simulink model "gm_HDL_pfc_gold_fi_vnl"  (R2024b)
settings: Solver=FixedStepDiscrete  StartTime=0.0  StopTime=.4  RelTol=1e-3
InitFcn:
  | fidelity_pfc_vals;
  | load('C:\Users\Angel\Desktop\hil\pfc3ph\matlab\sim\sschdl\pfc_desktop\stateSpaceParameters.mat');
undefined symbols (not defined in the file or in its folder): a, b, c, DiscIntNeverNeededParam, Down, Gs, s, stateSpaceParameters_1, t_ss, tsw, Up
libraries: simulink x32, hdlmdlgenlib x24, hdlsllib x8, eePwmGenerator x3, dspsrcs4 x3, hdlssclib x2, simulink_need_slupdate x1
(part 2 of 4)

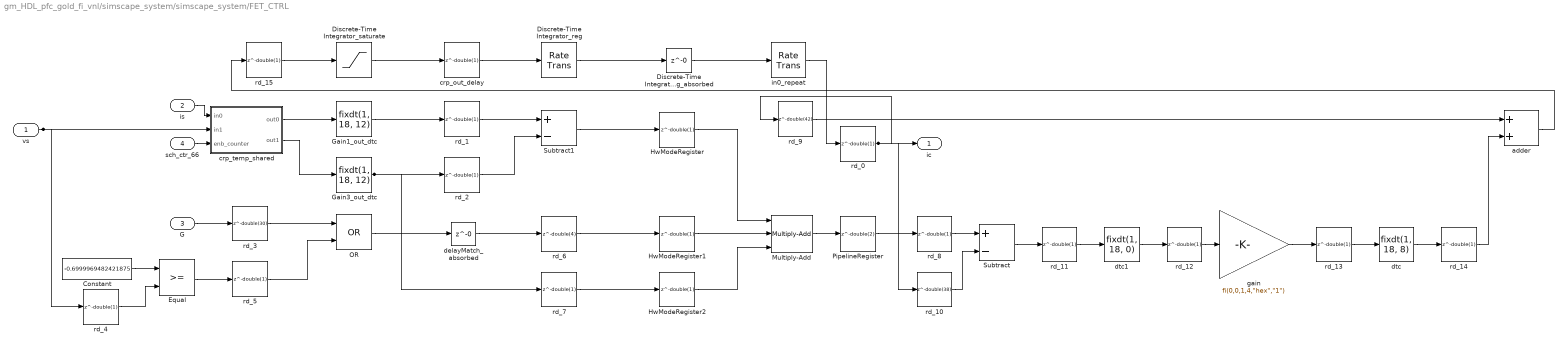
== system gm_HDL_pfc_gold_fi_vnl/simscape_system/simscape_system/FET_CTRL ==
  vs : Inport  OutDataTypeStr=fixdt(1, 18, 6)  PortDimensions=[6]  SampleTime=7.65403750478377e-09
  is : Inport  Port=2  OutDataTypeStr=fixdt(1, 18, 6)  PortDimensions=[6]  SampleTime=7.65403750478377e-09
  G : Inport  Port=3  OutDataTypeStr=boolean  PortDimensions=[6]  SampleTime=7.65403750478377e-09
  sch_ctr_66 : Inport  Port=4  OutDataTypeStr=fixdt(0, 7, 0)  SampleTime=7.65403750478377e-09
  Constant : Constant  Value=-0.6999969482421875  OutDataTypeStr=fixdt(1, 18, 17)  SampleTime=7.65403750478377e-09
  Discrete-Time Integrator_reg : RateTransition  InitialCondition=double(0)  OutPortSampleTimeOpt=Multiple of input port sample time  OutPortSampleTimeMultiple=67
  Discrete-Time Integrator_reg_absorbed : Delay  DelayLength=0
  Discrete-Time Integrator_saturate : Saturate  UpperLimit="fi(0,1,18,8,\"hex\",\"06400\")"  LowerLimit="fi(0,1,18,8,\"hex\",\"39c00\")"  SampleTime=7.65403750478377e-09  OutDataTypeStr=fixdt(1, 18, 8)
  Equal : RelationalOperator  OutDataTypeStr=boolean  SampleTime=7.65403750478377e-09  InputSameDT=off
  Gain1_out_dtc : DataTypeConversion  OutDataTypeStr=fixdt(1, 18, 12)  SampleTime=7.65403750478377e-09  SaturateOnIntegerOverflow=off  RndMeth=Floor
  Gain3_out_dtc : DataTypeConversion  OutDataTypeStr=fixdt(1, 18, 12)  SampleTime=7.65403750478377e-09  SaturateOnIntegerOverflow=off  RndMeth=Floor
  HwModeRegister : Delay  DelayLength=double(1)  InitialCondition=0  SampleTime=7.65403750478377e-09
  HwModeRegister1 : Delay  DelayLength=double(1)  InitialCondition=0  SampleTime=7.65403750478377e-09
  HwModeRegister2 : Delay  DelayLength=double(1)  InitialCondition=0  SampleTime=7.65403750478377e-09
  Multiply-Add : hdlsllib/HDL Operations/Multiply-Add  Function=c+(a.*b)  datatype=fixdt(1, 18, 12)  DoSatur=on  FMA=off
  OR : Logic  Operator=OR  AllPortsSameDT=off  OutDataTypeStr=boolean  SampleTime=7.65403750478377e-09
  PipelineRegister : Delay  DelayLength=double(2)  InitialCondition=0  SampleTime=7.65403750478377e-09
  Subtract : Sum  Inputs=+-  OutDataTypeStr=fixdt(1, 18, 12)  AccumDataTypeStr=fixdt(1, 23, 12)  SampleTime=7.65403750478377e-09
  Subtract1 : Sum  Inputs=+-  OutDataTypeStr=fixdt(1, 18, 11)  AccumDataTypeStr=fixdt(1, 19, 12)  SampleTime=7.65403750478377e-09
  adder : Sum  OutDataTypeStr=fixdt(1, 18, 8)  AccumDataTypeStr=fixdt(1, 18, 8)  SaturateOnIntegerOverflow=on  SampleTime=7.65403750478377e-09
  crp_out_delay : Delay  DelayLength=double(1)  InitialCondition=0  SampleTime=7.65403750478377e-09
  crp_temp_shared : Subsystem
  delayMatch_absorbed : Delay  DelayLength=0
  dtc : DataTypeConversion  OutDataTypeStr=fixdt(1, 18, 8)  ConvertRealWorld=Stored Integer (SI)  SampleTime=7.65403750478377e-09  RndMeth=Floor
  dtc1 : DataTypeConversion  OutDataTypeStr=fixdt(1, 18, 0)  ConvertRealWorld=Stored Integer (SI)  SampleTime=7.65403750478377e-09  RndMeth=Floor
  gain : Gain  Gain="fi(0,0,1,4,\"hex\",\"1\")"  ParamDataTypeStr=fixdt(0, 1, 4)  OutDataTypeStr=fixdt(1, 18, 0)  SaturateOnIntegerOverflow=on  SampleTime=7.65403750478377e-09
  in0_repeat : RateTransition  Integrity=off  Deterministic=off  OutPortSampleTimeOpt=Multiple of input port sample time  OutPortSampleTimeMultiple=1/67
  rd_{0..2,4..5,7..8,11..15} (12 alike) : Delay  DelayLength=double(1)  InitialCondition=0  SampleTime=7.65403750478377e-09
  rd_10 : Delay  DelayLength=double(38)  InitialCondition=0  SampleTime=7.65403750478377e-09
  rd_3 : Delay  DelayLength=double(30)  InitialCondition=0  SampleTime=7.65403750478377e-09
  rd_6 : Delay  DelayLength=double(4)  InitialCondition=0  SampleTime=7.65403750478377e-09
  rd_9 : Delay  DelayLength=double(42)  InitialCondition=0  SampleTime=7.65403750478377e-09
  ic : Outport  SampleTime=7.65403750478377e-09
  wires:
  adder/1 -> rd_15/1
  rd_14/1 -> adder/2
  rd_13/1 -> dtc/1
  dtc1/1 -> rd_12/1
  rd_8/1 -> Subtract/1
  PipelineRegister/1 -> rd_8/1
  rd_9/1 -> adder/1
  in0_repeat/1 -> rd_0/1
  HwModeRegister1/1 -> Multiply-Add/2
  rd_0/1 -> ic/1, rd_10/1, rd_9/1
  HwModeRegister/1 -> Multiply-Add/1
  Discrete-Time Integrator_reg_absorbed/1 -> in0_repeat/1
  gain/1 -> rd_13/1
  rd_7/1 -> HwModeRegister2/1
  rd_6/1 -> HwModeRegister1/1
  Multiply-Add/1 -> PipelineRegister/1
  delayMatch_absorbed/1 -> rd_6/1
  rd_2/1 -> Subtract1/2
  Discrete-Time Integrator_reg/1 -> Discrete-Time Integrator_reg_absorbed/1
  rd_1/1 -> Subtract1/1
  Subtract1/1 -> HwModeRegister/1
  crp_out_delay/1 -> Discrete-Time Integrator_reg/1
  Gain3_out_dtc/1 -> rd_2/1, rd_7/1
  Gain1_out_dtc/1 -> rd_1/1
  rd_11/1 -> dtc1/1
  Discrete-Time Integrator_saturate/1 -> crp_out_delay/1
  rd_5/1 -> OR/2
  dtc/1 -> rd_14/1
  rd_3/1 -> OR/1
  crp_temp_shared/2(out1) -> Gain3_out_dtc/1
  OR/1 -> delayMatch_absorbed/1
  Subtract/1 -> rd_11/1
  crp_temp_shared/1(out0) -> Gain1_out_dtc/1
  Equal/1 -> rd_5/1
  is/1 -> crp_temp_shared/1(in0)
  sch_ctr_66/1 -> crp_temp_shared/3(enb_counter)
  G/1 -> rd_3/1
  rd_12/1 -> gain/1
  rd_4/1 -> Equal/2
  Constant/1 -> Equal/1
  HwModeRegister2/1 -> Multiply-Add/3
  rd_15/1 -> Discrete-Time Integrator_saturate/1
  vs/1 -> rd_4/1, crp_temp_shared/2(in1)
  rd_10/1 -> Subtract/2

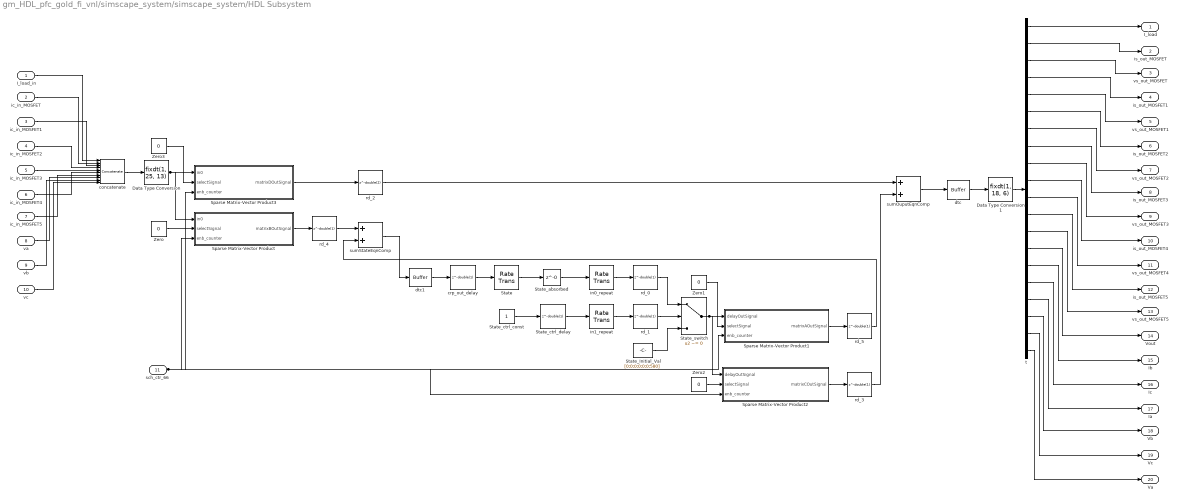
== system gm_HDL_pfc_gold_fi_vnl/simscape_system/simscape_system/HDL Subsystem ==
  I_load_in : Inport  OutDataTypeStr=fixdt(1, 18, 8)  PortDimensions=1  SampleTime=7.65403750478377e-09
  ic_in_MOSFET : Inport  Port=2  OutDataTypeStr=fixdt(1, 18, 8)  PortDimensions=1  SampleTime=7.65403750478377e-09
  ic_in_MOSFET1 : Inport  Port=3  OutDataTypeStr=fixdt(1, 18, 8)  PortDimensions=1  SampleTime=7.65403750478377e-09
  ic_in_MOSFET2 : Inport  Port=4  OutDataTypeStr=fixdt(1, 18, 8)  PortDimensions=1  SampleTime=7.65403750478377e-09
  ic_in_MOSFET3 : Inport  Port=5  OutDataTypeStr=fixdt(1, 18, 8)  PortDimensions=1  SampleTime=7.65403750478377e-09
  ic_in_MOSFET4 : Inport  Port=6  OutDataTypeStr=fixdt(1, 18, 8)  PortDimensions=1  SampleTime=7.65403750478377e-09
  ic_in_MOSFET5 : Inport  Port=7  OutDataTypeStr=fixdt(1, 18, 8)  PortDimensions=1  SampleTime=7.65403750478377e-09
  va : Inport  Port=8  OutDataTypeStr=fixdt(1, 18, 8)  PortDimensions=1  SampleTime=7.65403750478377e-09
  vb : Inport  Port=9  OutDataTypeStr=fixdt(1, 18, 8)  PortDimensions=1  SampleTime=7.65403750478377e-09
  vc : Inport  Port=10  OutDataTypeStr=fixdt(1, 18, 8)  PortDimensions=1  SampleTime=7.65403750478377e-09
  sch_ctr_66 : Inport  Port=11  OutDataTypeStr=fixdt(0, 7, 0)  SampleTime=7.65403750478377e-09
  Data Type Conversion : DataTypeConversion  OutDataTypeStr=fixdt(1, 25, 13)  SampleTime=7.65403750478377e-09  SaturateOnIntegerOverflow=off  RndMeth=Floor
  Data Type Conversion1 : DataTypeConversion  OutDataTypeStr=fixdt(1, 18, 6)  SampleTime=7.65403750478377e-09  SaturateOnIntegerOverflow=off  RndMeth=Floor
  Sparse Matrix-Vector Product : Subsystem
  Sparse Matrix-Vector Product1 : Subsystem
  Sparse Matrix-Vector Product2 : Subsystem
  Sparse Matrix-Vector Product3 : Subsystem
  State : RateTransition  InitialCondition=double(0)  OutPortSampleTimeOpt=Multiple of input port sample time  OutPortSampleTimeMultiple=67
  State_Initial_Val : Constant  Value=[0;0;0;0;0;0;580]  OutDataTypeStr=fixdt(1, 25, 13)  SampleTime=7.65403750478377e-09
  State_absorbed : Delay  DelayLength=0
  State_ctrl_const : Constant  OutDataTypeStr=boolean  SampleTime=5.12820512820513e-07
  State_ctrl_delay : Delay  DelayLength=double(1)  InitialCondition=0  SampleTime=5.12820512820513e-07
  State_switch : Switch  Criteria=u2 ~= 0  Threshold=double(0)  OutDataTypeStr=fixdt(1, 25, 13)  SampleTime=7.65403750478377e-09  SaturateOnIntegerOverflow=off  InputSameDT=off
  Zero{,1..3} (4 alike) : Constant  Value=0  OutDataTypeStr=boolean  SampleTime=7.65403750478377e-09
  concatenate : Concatenate  NumInputs=10
  crp_out_delay : Delay  DelayLength=double(1)  InitialCondition=0  SampleTime=7.65403750478377e-09
  dtc : hdlmdlgenlib/Buffer
  dtc1 : hdlmdlgenlib/Buffer
  in0_repeat : RateTransition  Integrity=off  Deterministic=off  OutPortSampleTimeOpt=Multiple of input port sample time  OutPortSampleTimeMultiple=1/67
  in1_repeat : RateTransition  Integrity=off  Deterministic=off  OutPortSampleTimeOpt=Multiple of input port sample time  OutPortSampleTimeMultiple=1/67
  rd_{0..1,3..5} (5 alike) : Delay  DelayLength=double(1)  InitialCondition=0  SampleTime=7.65403750478377e-09
  rd_2 : Delay  DelayLength=double(2)  InitialCondition=0  SampleTime=7.65403750478377e-09
  sumOuputEqnComp : Sum  OutDataTypeStr=fixdt(1, 25, 13)  SampleTime=7.65403750478377e-09
  sumStateEqnComp : Sum  OutDataTypeStr=fixdt(1, 25, 13)  SampleTime=7.65403750478377e-09
  t : Demux  Outputs=20
  I_load : Outport  SampleTime=7.65403750478377e-09
  is_out_MOSFET : Outport  Port=2  SampleTime=7.65403750478377e-09
  vs_out_MOSFET : Outport  Port=3  SampleTime=7.65403750478377e-09
  is_out_MOSFET1 : Outport  Port=4  SampleTime=7.65403750478377e-09
  vs_out_MOSFET1 : Outport  Port=5  SampleTime=7.65403750478377e-09
  is_out_MOSFET2 : Outport  Port=6  SampleTime=7.65403750478377e-09
  vs_out_MOSFET2 : Outport  Port=7  SampleTime=7.65403750478377e-09
  is_out_MOSFET3 : Outport  Port=8  SampleTime=7.65403750478377e-09
  vs_out_MOSFET3 : Outport  Port=9  SampleTime=7.65403750478377e-09
  is_out_MOSFET4 : Outport  Port=10  SampleTime=7.65403750478377e-09
  vs_out_MOSFET4 : Outport  Port=11  SampleTime=7.65403750478377e-09
  is_out_MOSFET5 : Outport  Port=12  SampleTime=7.65403750478377e-09
  vs_out_MOSFET5 : Outport  Port=13  SampleTime=7.65403750478377e-09
  Vout : Outport  Port=14  SampleTime=7.65403750478377e-09
  Ib : Outport  Port=15  SampleTime=7.65403750478377e-09
  Ic : Outport  Port=16  SampleTime=7.65403750478377e-09
  Ia : Outport  Port=17  SampleTime=7.65403750478377e-09
  Vb : Outport  Port=18  SampleTime=7.65403750478377e-09
  Vc : Outport  Port=19  SampleTime=7.65403750478377e-09
  Va : Outport  Port=20  SampleTime=7.65403750478377e-09
  wires:
  t/19 -> Vc/1
  t/18 -> Vb/1
  t/17 -> Ia/1
  t/14 -> Vout/1
  t/12 -> is_out_MOSFET5/1
  t/8 -> is_out_MOSFET3/1
  t/5 -> vs_out_MOSFET1/1
  t/4 -> is_out_MOSFET1/1
  t/3 -> vs_out_MOSFET/1
  t/2 -> is_out_MOSFET/1
  dtc/1 -> Data Type Conversion1/1
  rd_3/1 -> sumOuputEqnComp/2
  t/6 -> is_out_MOSFET2/1
  rd_5/1 -> sumStateEqnComp/2
  Data Type Conversion1/1 -> t/1
  Zero2/1 -> Sparse Matrix-Vector Product2/2(selectSignal)
  State_switch/1 -> Sparse Matrix-Vector Product2/1(delayOutSignal), Sparse Matrix-Vector Product1/1(delayOutSignal)
  Sparse Matrix-Vector Product1/1(matrixAOutSignal) -> rd_5/1
  State_Initial_Val/1 -> State_switch/3
  t/7 -> vs_out_MOSFET2/1
  in0_repeat/1 -> rd_0/1
  State_ctrl_delay/1 -> in1_repeat/1
  Zero1/1 -> Sparse Matrix-Vector Product1/2(selectSignal)
  State_absorbed/1 -> in0_repeat/1
  State_ctrl_const/1 -> State_ctrl_delay/1
  dtc1/1 -> crp_out_delay/1
  sumOuputEqnComp/1 -> dtc/1
  t/11 -> vs_out_MOSFET4/1
  sumStateEqnComp/1 -> dtc1/1
  rd_0/1 -> State_switch/1
  rd_2/1 -> sumOuputEqnComp/1
  rd_4/1 -> sumStateEqnComp/1
  in1_repeat/1 -> rd_1/1
  Sparse Matrix-Vector Product/1(matrixBOutSignal) -> rd_4/1
  Sparse Matrix-Vector Product3/1(matrixDOutSignal) -> rd_2/1
  sch_ctr_66/1 -> Sparse Matrix-Vector Product/3(enb_counter), Sparse Matrix-Vector Product3/3(enb_counter), Sparse Matrix-Vector Product1/3(enb_counter), Sparse Matrix-Vector Product2/3(enb_counter)
  t/15 -> Ib/1
  t/20 -> Va/1
  Zero/1 -> Sparse Matrix-Vector Product/2(selectSignal)
  rd_1/1 -> State_switch/2
  Zero3/1 -> Sparse Matrix-Vector Product3/2(selectSignal)
  t/10 -> is_out_MOSFET4/1
  concatenate/1 -> Data Type Conversion/1
  vc/1 -> concatenate/10
  t/9 -> vs_out_MOSFET3/1
  t/13 -> vs_out_MOSFET5/1
  vb/1 -> concatenate/9
  State/1 -> State_absorbed/1
  va/1 -> concatenate/8
  ic_in_MOSFET5/1 -> concatenate/7
  Sparse Matrix-Vector Product2/1(matrixCOutSignal) -> rd_3/1
  t/16 -> Ic/1
  ic_in_MOSFET2/1 -> concatenate/4
  Data Type Conversion/1 -> Sparse Matrix-Vector Product/1(in0), Sparse Matrix-Vector Product3/1(in0)
  ic_in_MOSFET1/1 -> concatenate/3
  ic_in_MOSFET/1 -> concatenate/2
  t/1 -> I_load/1
  ic_in_MOSFET4/1 -> concatenate/6
  crp_out_delay/1 -> State/1
  I_load_in/1 -> concatenate/1
  ic_in_MOSFET3/1 -> concatenate/5

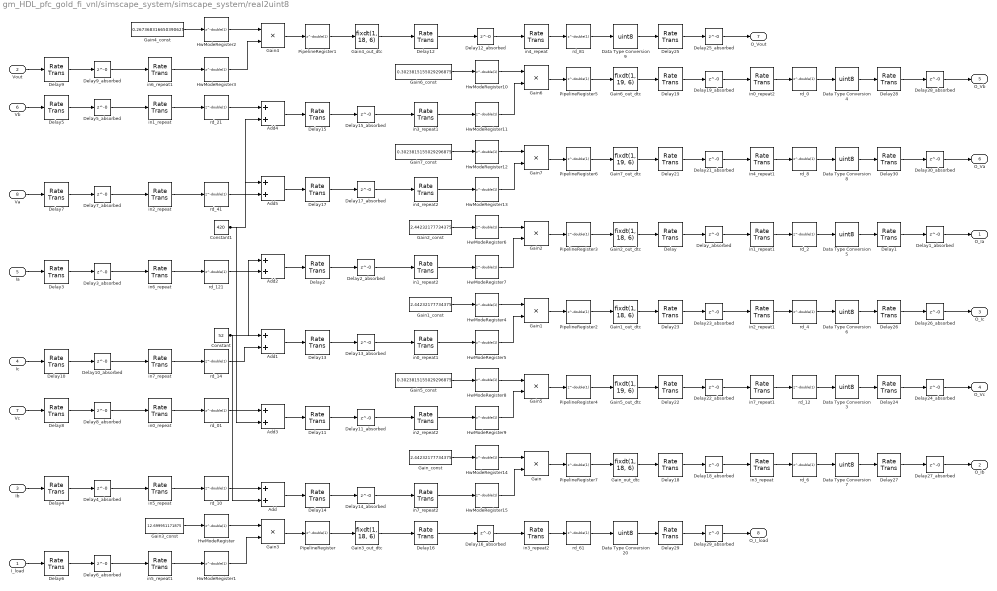
== system gm_HDL_pfc_gold_fi_vnl/simscape_system/simscape_system/real2uint8 ==
  I_load : Inport  OutDataTypeStr=fixdt(1, 18, 6)  PortDimensions=1  SampleTime=7.65403750478377e-09
  Vout : Inport  Port=2  OutDataTypeStr=fixdt(1, 18, 6)  PortDimensions=1  SampleTime=7.65403750478377e-09
  Ib : Inport  Port=3  OutDataTypeStr=fixdt(1, 18, 6)  PortDimensions=1  SampleTime=7.65403750478377e-09
  Ic : Inport  Port=4  OutDataTypeStr=fixdt(1, 18, 6)  PortDimensions=1  SampleTime=7.65403750478377e-09
  Ia : Inport  Port=5  OutDataTypeStr=fixdt(1, 18, 6)  PortDimensions=1  SampleTime=7.65403750478377e-09
  Vb : Inport  Port=6  OutDataTypeStr=fixdt(1, 18, 6)  PortDimensions=1  SampleTime=7.65403750478377e-09
  Vc : Inport  Port=7  OutDataTypeStr=fixdt(1, 18, 6)  PortDimensions=1  SampleTime=7.65403750478377e-09
  Va : Inport  Port=8  OutDataTypeStr=fixdt(1, 18, 6)  PortDimensions=1  SampleTime=7.65403750478377e-09
  Add : Sum  OutDataTypeStr=fixdt(1, 18, 6)  AccumDataTypeStr=fixdt(1, 19, 6)  SampleTime=7.65403750478377e-09
  Add1 : Sum  OutDataTypeStr=fixdt(1, 18, 6)  AccumDataTypeStr=fixdt(1, 19, 6)  SampleTime=7.65403750478377e-09
  Add2 : Sum  OutDataTypeStr=fixdt(1, 18, 6)  AccumDataTypeStr=fixdt(1, 19, 6)  SampleTime=7.65403750478377e-09
  Add3 : Sum  OutDataTypeStr=fixdt(1, 19, 6)  AccumDataTypeStr=fixdt(1, 19, 6)  SampleTime=7.65403750478377e-09
  Add4 : Sum  OutDataTypeStr=fixdt(1, 19, 6)  AccumDataTypeStr=fixdt(1, 19, 6)  SampleTime=7.65403750478377e-09
  Add5 : Sum  OutDataTypeStr=fixdt(1, 19, 6)  AccumDataTypeStr=fixdt(1, 19, 6)  SampleTime=7.65403750478377e-09
  Constant : Constant  Value=52  OutDataTypeStr=fixdt(1, 18, 6)  SampleTime=7.65403750478377e-09
  Constant1 : Constant  Value=420  OutDataTypeStr=fixdt(1, 18, 6)  SampleTime=7.65403750478377e-09
  Data Type Conversion{3..9,20} (8 alike) : DataTypeConversion  OutDataTypeStr=uint8  RndMeth=Nearest  SampleTime=7.65403750478377e-09  SaturateOnIntegerOverflow=off
  Delay{,1..19,21..30} (30 alike) : RateTransition  InitialCondition=double(0)  OutPortSampleTimeOpt=Multiple of input port sample time  OutPortSampleTimeMultiple=67
  Delay10_absorbed : Delay  DelayLength=0
  Delay11_absorbed : Delay  DelayLength=0
  Delay12_absorbed : Delay  DelayLength=0
  Delay13_absorbed : Delay  DelayLength=0
  Delay14_absorbed : Delay  DelayLength=0
  Delay15_absorbed : Delay  DelayLength=0
  Delay16_absorbed : Delay  DelayLength=0
  Delay17_absorbed : Delay  DelayLength=0
  Delay18_absorbed : Delay  DelayLength=0
  Delay19_absorbed : Delay  DelayLength=0
  Delay1_absorbed : Delay  DelayLength=0
  Delay21_absorbed : Delay  DelayLength=0
  Delay22_absorbed : Delay  DelayLength=0
  Delay23_absorbed : Delay  DelayLength=0
  Delay24_absorbed : Delay  DelayLength=0
  Delay25_absorbed : Delay  DelayLength=0
  Delay26_absorbed : Delay  DelayLength=0
  Delay27_absorbed : Delay  DelayLength=0
  Delay28_absorbed : Delay  DelayLength=0
  Delay29_absorbed : Delay  DelayLength=0
  Delay2_absorbed : Delay  DelayLength=0
  Delay30_absorbed : Delay  DelayLength=0
  Delay3_absorbed : Delay  DelayLength=0
  Delay4_absorbed : Delay  DelayLength=0
  Delay5_absorbed : Delay  DelayLength=0
  Delay6_absorbed : Delay  DelayLength=0
  Delay7_absorbed : Delay  DelayLength=0
  Delay8_absorbed : Delay  DelayLength=0
  Delay9_absorbed : Delay  DelayLength=0
  Delay_absorbed : Delay  DelayLength=0
  Gain : Product  Inputs=**  OutDataTypeStr=fixdt(1, 36, 21)  SampleTime=7.65403750478377e-09
  Gain1 : Product  Inputs=**  OutDataTypeStr=fixdt(1, 36, 21)  SampleTime=7.65403750478377e-09
  Gain1_const : Constant  Value=2.44232177734375  OutDataTypeStr=fixdt(1, 18, 15)  SampleTime=7.65403750478377e-09
  Gain1_out_dtc : DataTypeConversion  OutDataTypeStr=fixdt(1, 18, 6)  SampleTime=7.65403750478377e-09  SaturateOnIntegerOverflow=off  RndMeth=Floor
  Gain2 : Product  Inputs=**  OutDataTypeStr=fixdt(1, 36, 21)  SampleTime=7.65403750478377e-09
  Gain2_const : Constant  Value=2.44232177734375  OutDataTypeStr=fixdt(1, 18, 15)  SampleTime=7.65403750478377e-09
  Gain2_out_dtc : DataTypeConversion  OutDataTypeStr=fixdt(1, 18, 6)  SampleTime=7.65403750478377e-09  SaturateOnIntegerOverflow=off  RndMeth=Floor
  Gain3 : Product  Inputs=**  OutDataTypeStr=fixdt(1, 36, 19)  SampleTime=7.65403750478377e-09
  Gain3_const : Constant  Value=12.699951171875  OutDataTypeStr=fixdt(1, 18, 13)  SampleTime=7.65403750478377e-09
  Gain3_out_dtc : DataTypeConversion  OutDataTypeStr=fixdt(1, 18, 6)  SampleTime=7.65403750478377e-09  SaturateOnIntegerOverflow=off  RndMeth=Floor
  Gain4 : Product  Inputs=**  OutDataTypeStr=fixdt(1, 36, 24)  SampleTime=7.65403750478377e-09
  Gain4_const : Constant  Value=0.267368316650390625  OutDataTypeStr=fixdt(1, 18, 18)  SampleTime=7.65403750478377e-09
  Gain4_out_dtc : DataTypeConversion  OutDataTypeStr=fixdt(1, 18, 6)  SampleTime=7.65403750478377e-09  SaturateOnIntegerOverflow=off  RndMeth=Floor
  Gain5 : Product  Inputs=**  OutDataTypeStr=fixdt(1, 38, 25)  SampleTime=7.65403750478377e-09
  Gain5_const : Constant  Value=0.3023815155029296875  OutDataTypeStr=fixdt(1, 19, 19)  SampleTime=7.65403750478377e-09
  Gain5_out_dtc : DataTypeConversion  OutDataTypeStr=fixdt(1, 19, 6)  SampleTime=7.65403750478377e-09  SaturateOnIntegerOverflow=off  RndMeth=Floor
  Gain6 : Product  Inputs=**  OutDataTypeStr=fixdt(1, 38, 25)  SampleTime=7.65403750478377e-09
  Gain6_const : Constant  Value=0.3023815155029296875  OutDataTypeStr=fixdt(1, 19, 19)  SampleTime=7.65403750478377e-09
  Gain6_out_dtc : DataTypeConversion  OutDataTypeStr=fixdt(1, 19, 6)  SampleTime=7.65403750478377e-09  SaturateOnIntegerOverflow=off  RndMeth=Floor
  Gain7 : Product  Inputs=**  OutDataTypeStr=fixdt(1, 38, 25)  SampleTime=7.65403750478377e-09
  Gain7_const : Constant  Value=0.3023815155029296875  OutDataTypeStr=fixdt(1, 19, 19)  SampleTime=7.65403750478377e-09
  Gain7_out_dtc : DataTypeConversion  OutDataTypeStr=fixdt(1, 19, 6)  SampleTime=7.65403750478377e-09  SaturateOnIntegerOverflow=off  RndMeth=Floor
  Gain_const : Constant  Value=2.44232177734375  OutDataTypeStr=fixdt(1, 18, 15)  SampleTime=7.65403750478377e-09
  Gain_out_dtc : DataTypeConversion  OutDataTypeStr=fixdt(1, 18, 6)  SampleTime=7.65403750478377e-09  SaturateOnIntegerOverflow=off  RndMeth=Floor
  HwModeRegister{,1..15} (16 alike) : Delay  DelayLength=double(1)  InitialCondition=0  SampleTime=7.65403750478377e-09
  PipelineRegister{,1..7} (8 alike) : Delay  DelayLength=double(1)  InitialCondition=0  SampleTime=7.65403750478377e-09
  in0_repeat : RateTransition  Integrity=off  Deterministic=off  OutPortSampleTimeOpt=Multiple of input port sample time  OutPortSampleTimeMultiple=1/67
  in0_repeat1 : RateTransition  Integrity=off  Deterministic=off  OutPortSampleTimeOpt=Multiple of input port sample time  OutPortSampleTimeMultiple=1/67
  in0_repeat2 : RateTransition  Integrity=off  Deterministic=off  OutPortSampleTimeOpt=Multiple of input port sample time  OutPortSampleTimeMultiple=1/67
  in1_repeat : RateTransition  Integrity=off  Deterministic=off  OutPortSampleTimeOpt=Multiple of input port sample time  OutPortSampleTimeMultiple=1/67
  in1_repeat1 : RateTransition  Integrity=off  Deterministic=off  OutPortSampleTimeOpt=Multiple of input port sample time  OutPortSampleTimeMultiple=1/67
  in1_repeat2 : RateTransition  Integrity=off  Deterministic=off  OutPortSampleTimeOpt=Multiple of input port sample time  OutPortSampleTimeMultiple=1/67
  in2_repeat : RateTransition  Integrity=off  Deterministic=off  OutPortSampleTimeOpt=Multiple of input port sample time  OutPortSampleTimeMultiple=1/67
  in2_repeat1 : RateTransition  Integrity=off  Deterministic=off  OutPortSampleTimeOpt=Multiple of input port sample time  OutPortSampleTimeMultiple=1/67
  in2_repeat2 : RateTransition  Integrity=off  Deterministic=off  OutPortSampleTimeOpt=Multiple of input port sample time  OutPortSampleTimeMultiple=1/67
  in3_repeat : RateTransition  Integrity=off  Deterministic=off  OutPortSampleTimeOpt=Multiple of input port sample time  OutPortSampleTimeMultiple=1/67
  in3_repeat1 : RateTransition  Integrity=off  Deterministic=off  OutPortSampleTimeOpt=Multiple of input port sample time  OutPortSampleTimeMultiple=1/67
  in3_repeat2 : RateTransition  Integrity=off  Deterministic=off  OutPortSampleTimeOpt=Multiple of input port sample time  OutPortSampleTimeMultiple=1/67
  in4_repeat : RateTransition  Integrity=off  Deterministic=off  OutPortSampleTimeOpt=Multiple of input port sample time  OutPortSampleTimeMultiple=1/67
  in4_repeat1 : RateTransition  Integrity=off  Deterministic=off  OutPortSampleTimeOpt=Multiple of input port sample time  OutPortSampleTimeMultiple=1/67
  in4_repeat2 : RateTransition  Integrity=off  Deterministic=off  OutPortSampleTimeOpt=Multiple of input port sample time  OutPortSampleTimeMultiple=1/67
  in5_repeat : RateTransition  Integrity=off  Deterministic=off  OutPortSampleTimeOpt=Multiple of input port sample time  OutPortSampleTimeMultiple=1/67
  in5_repeat1 : RateTransition  Integrity=off  Deterministic=off  OutPortSampleTimeOpt=Multiple of input port sample time  OutPortSampleTimeMultiple=1/67
  in6_repeat : RateTransition  Integrity=off  Deterministic=off  OutPortSampleTimeOpt=Multiple of input port sample time  OutPortSampleTimeMultiple=1/67
  in6_repeat1 : RateTransition  Integrity=off  Deterministic=off  OutPortSampleTimeOpt=Multiple of input port sample time  OutPortSampleTimeMultiple=1/67
  in7_repeat : RateTransition  Integrity=off  Deterministic=off  OutPortSampleTimeOpt=Multiple of input port sample time  OutPortSampleTimeMultiple=1/67
  in7_repeat1 : RateTransition  Integrity=off  Deterministic=off  OutPortSampleTimeOpt=Multiple of input port sample time  OutPortSampleTimeMultiple=1/67
  in7_repeat2 : RateTransition  Integrity=off  Deterministic=off  OutPortSampleTimeOpt=Multiple of input port sample time  OutPortSampleTimeMultiple=1/67
  rd_{0,2,4,6,8,10,12,14,21,41,61,81,121} (13 alike) : Delay  DelayLength=double(1)  InitialCondition=0  SampleTime=7.65403750478377e-09
  rd_01 : Delay  DelayLength=double(1)  InitialCondition=0  SampleTime=7.65403750478377e-09
  O_Ia : Outport  SampleTime=5.12820512820513e-07
  O_Ib : Outport  Port=2  SampleTime=5.12820512820513e-07
  O_Ic : Outport  Port=3  SampleTime=5.12820512820513e-07
  O_Vc : Outport  Port=4  SampleTime=5.12820512820513e-07
  O_Vb : Outport  Port=5  SampleTime=5.12820512820513e-07
  O_Va : Outport  Port=6  SampleTime=5.12820512820513e-07
  O_Vout : Outport  Port=7  SampleTime=5.12820512820513e-07
  O_I_load : Outport  Port=8  SampleTime=5.12820512820513e-07
  wires:
  Ib/1 -> Delay4/1
  Ia/1 -> Delay3/1
  Vb/1 -> Delay5/1
  Data Type Conversion9/1 -> Delay25/1
  Delay29_absorbed/1 -> O_I_load/1
  Delay25_absorbed/1 -> O_Vout/1
  Data Type Conversion4/1 -> Delay28/1
  Data Type Conversion5/1 -> Delay1/1
  Data Type Conversion6/1 -> Delay26/1
  Data Type Conversion7/1 -> Delay27/1
  Data Type Conversion3/1 -> Delay24/1
  Delay1/1 -> Delay1_absorbed/1
  Delay28/1 -> Delay28_absorbed/1
  Delay30/1 -> Delay30_absorbed/1
  Delay24/1 -> Delay24_absorbed/1
  Delay1_absorbed/1 -> O_Ia/1
  Delay26_absorbed/1 -> O_Ic/1
  Delay27_absorbed/1 -> O_Ib/1
  Delay24_absorbed/1 -> O_Vc/1
  Data Type Conversion20/1 -> Delay29/1
  Delay29/1 -> Delay29_absorbed/1
  Delay4/1 -> Delay4_absorbed/1
  Delay5/1 -> Delay5_absorbed/1
  Delay7/1 -> Delay7_absorbed/1
  Delay4_absorbed/1 -> in5_repeat/1
  Delay5_absorbed/1 -> in1_repeat/1
  Delay7_absorbed/1 -> in2_repeat/1
  Delay8_absorbed/1 -> in0_repeat/1
  Delay28_absorbed/1 -> O_Vb/1
  Va/1 -> Delay7/1
  Add3/1 -> Delay11/1
  Add5/1 -> Delay17/1
  Add2/1 -> Delay2/1
  Add1/1 -> Delay13/1
  in1_repeat/1 -> rd_21/1
  in6_repeat/1 -> rd_121/1
  in7_repeat/1 -> rd_14/1
  I_load/1 -> Delay6/1
  in4_repeat/1 -> rd_81/1
  in3_repeat2/1 -> rd_61/1
  Delay12/1 -> Delay12_absorbed/1
  Add4/1 -> Delay15/1
  Delay12_absorbed/1 -> in4_repeat/1
  Gain4_out_dtc/1 -> Delay12/1
  Delay22_absorbed/1 -> in7_repeat1/1
  Gain1_out_dtc/1 -> Delay23/1
  Gain2_out_dtc/1 -> Delay/1
  Gain5_out_dtc/1 -> Delay22/1
  Gain6_out_dtc/1 -> Delay19/1
  Delay9_absorbed/1 -> in6_repeat1/1
  in0_repeat/1 -> rd_01/1
  in6_repeat1/1 -> HwModeRegister3/1
  Delay6/1 -> Delay6_absorbed/1
  in5_repeat1/1 -> HwModeRegister1/1
  Delay21/1 -> Delay21_absorbed/1
  Delay30_absorbed/1 -> O_Va/1
  Delay21_absorbed/1 -> in4_repeat1/1
  in4_repeat1/1 -> rd_8/1
  Delay10/1 -> Delay10_absorbed/1
  Delay18/1 -> Delay18_absorbed/1
  Delay18_absorbed/1 -> in3_repeat/1
  in3_repeat/1 -> rd_6/1
  Delay23/1 -> Delay23_absorbed/1
  Ic/1 -> Delay10/1
  Delay23_absorbed/1 -> in2_repeat1/1
  in2_repeat1/1 -> rd_4/1
  in1_repeat1/1 -> rd_2/1
  Constant1/1 -> Add3/2, Add4/2, Add5/1
  Add/1 -> Delay14/1
  Delay14/1 -> Delay14_absorbed/1
  in7_repeat2/1 -> HwModeRegister15/1
  Delay6_absorbed/1 -> in5_repeat1/1
  Delay17_absorbed/1 -> in4_repeat2/1
  in4_repeat2/1 -> HwModeRegister13/1
  Delay15/1 -> Delay15_absorbed/1
  Delay15_absorbed/1 -> in3_repeat1/1
  in3_repeat1/1 -> HwModeRegister11/1
  Delay11/1 -> Delay11_absorbed/1
  Delay27/1 -> Delay27_absorbed/1
  Delay11_absorbed/1 -> in2_repeat2/1
  Delay/1 -> Delay_absorbed/1
  in5_repeat/1 -> rd_10/1
  in2_repeat2/1 -> HwModeRegister9/1
  Delay2_absorbed/1 -> in1_repeat2/1
  Delay13_absorbed/1 -> in0_repeat1/1
  in0_repeat1/1 -> HwModeRegister5/1
  Delay16_absorbed/1 -> in3_repeat2/1
  Gain3_const/1 -> HwModeRegister/1
  in2_repeat/1 -> rd_41/1
  rd_6/1 -> Data Type Conversion7/1
  Delay3/1 -> Delay3_absorbed/1
  PipelineRegister2/1 -> Gain1_out_dtc/1
  Gain_out_dtc/1 -> Delay18/1
  PipelineRegister4/1 -> Gain5_out_dtc/1
  rd_81/1 -> Data Type Conversion9/1
  Gain7_out_dtc/1 -> Delay21/1
  PipelineRegister7/1 -> Gain_out_dtc/1
  Delay26/1 -> Delay26_absorbed/1
  rd_41/1 -> Add5/2
  rd_10/1 -> Add/1
  Data Type Conversion8/1 -> Delay30/1
  Delay13/1 -> Delay13_absorbed/1
  Delay19/1 -> Delay19_absorbed/1
  Gain3/1 -> PipelineRegister/1
  HwModeRegister/1 -> Gain3/1
  Gain7_const/1 -> HwModeRegister12/1
  Delay14_absorbed/1 -> in7_repeat2/1
  Delay16/1 -> Delay16_absorbed/1
  rd_61/1 -> Data Type Conversion20/1
  Delay25/1 -> Delay25_absorbed/1
  PipelineRegister5/1 -> Gain6_out_dtc/1
  HwModeRegister1/1 -> Gain3/2
  Delay22/1 -> Delay22_absorbed/1
  Vout/1 -> Delay9/1
  Gain5_const/1 -> HwModeRegister8/1
  Gain3_out_dtc/1 -> Delay16/1
  Gain4/1 -> PipelineRegister1/1
  HwModeRegister3/1 -> Gain4/2
  Gain_const/1 -> HwModeRegister14/1
  rd_01/1 -> Add3/1
  rd_121/1 -> Add2/2
  HwModeRegister4/1 -> Gain1/1
  in7_repeat1/1 -> rd_12/1
  Gain2/1 -> PipelineRegister3/1
  rd_4/1 -> Data Type Conversion6/1
  PipelineRegister1/1 -> Gain4_out_dtc/1
  rd_2/1 -> Data Type Conversion5/1
  HwModeRegister7/1 -> Gain2/2
  in0_repeat2/1 -> rd_0/1
  Gain5/1 -> PipelineRegister4/1
  rd_14/1 -> Add1/2
  Delay17/1 -> Delay17_absorbed/1
  Delay19_absorbed/1 -> in0_repeat2/1
  Delay3_absorbed/1 -> in6_repeat/1
  Gain1_const/1 -> HwModeRegister4/1
  rd_0/1 -> Data Type Conversion4/1
  PipelineRegister/1 -> Gain3_out_dtc/1
  Gain6_const/1 -> HwModeRegister10/1
  Vc/1 -> Delay8/1
  Gain6/1 -> PipelineRegister5/1
  Delay9/1 -> Delay9_absorbed/1
  rd_8/1 -> Data Type Conversion8/1
  HwModeRegister2/1 -> Gain4/1
  PipelineRegister6/1 -> Gain7_out_dtc/1
  HwModeRegister8/1 -> Gain5/1
  HwModeRegister5/1 -> Gain1/2
  HwModeRegister12/1 -> Gain7/1
  in1_repeat2/1 -> HwModeRegister7/1
  Delay_absorbed/1 -> in1_repeat1/1
  HwModeRegister13/1 -> Gain7/2
  Delay10_absorbed/1 -> in7_repeat/1
  HwModeRegister9/1 -> Gain5/2
  Gain7/1 -> PipelineRegister6/1
  Delay8/1 -> Delay8_absorbed/1
  PipelineRegister3/1 -> Gain2_out_dtc/1
  Gain1/1 -> PipelineRegister2/1
  Gain/1 -> PipelineRegister7/1
  HwModeRegister14/1 -> Gain/1
  Constant/1 -> Add2/1, Add1/1, Add/2
  HwModeRegister6/1 -> Gain2/1
  HwModeRegister11/1 -> Gain6/2
  Delay2/1 -> Delay2_absorbed/1
  rd_21/1 -> Add4/1
  rd_12/1 -> Data Type Conversion3/1
  HwModeRegister15/1 -> Gain/2
  HwModeRegister10/1 -> Gain6/1
  Gain2_const/1 -> HwModeRegister6/1
  Gain4_const/1 -> HwModeRegister2/1

== system gm_HDL_pfc_gold_fi_vnl/simscape_system_vnl/HDL Subsystem/HDL Algorithm ==
  In1 : Inport
  Delay1 : Delay  DelayLength=1
  Delay2 : Delay
  Output : Subsystem
  Sel : Constant  Value=0  OutDataTypeStr=uint32  SampleTime=-1
  State Delay : Delay  DelayLength=1  InitialCondition=single(stateSpaceParameters_1.X0)
  State Switch : Switch  Criteria=u2 ~= 0  SaturateOnIntegerOverflow=off  InputSameDT=off
  State Update : Subsystem
  Valid Out : Constant  OutDataTypeStr=boolean  SampleTime=4.395604395604395e-07
  X0 : Constant  Value=single(stateSpaceParameters_1.X0)  SampleTime=4.395604395604395e-07
  Out1 : Outport  VectorParamsAs1DForOutWhenUnconnected=off
  wires:
  In1/1 -> State Update/1(In1), Delay1/1
  State Switch/1 -> State Update/2(State), Output/2(State)
  Output/1(Out1) -> Out1/1
  X0/1 -> State Switch/3
  Delay2/1 -> State Switch/2
  State Delay/1 -> State Switch/1
  Valid Out/1 -> Delay2/1
  State Update/1(State Out) -> State Delay/1
  Sel/1 -> State Update/3(Sel), Output/3(Sel)
  Delay1/1 -> Output/1(In1)

== system gm_HDL_pfc_gold_fi_vnl/simscape_system/simscape_system/FET_CTRL/crp_temp_shared ==
  in0 : Inport  OutDataTypeStr=fixdt(1, 18, 6)  PortDimensions=[6]  SampleTime=7.65403750478377e-09
  in1 : Inport  Port=2  OutDataTypeStr=fixdt(1, 18, 6)  PortDimensions=[6]  SampleTime=7.65403750478377e-09
  enb_counter : Inport  Port=3  OutDataTypeStr=fixdt(0, 7, 0)  SampleTime=7.65403750478377e-09
  Gain1 : Product  Inputs=**  OutDataTypeStr=fixdt(1, 36, 0)  SampleTime=7.65403750478377e-09
  Gain1_const : Constant  Value=-1  OutDataTypeStr=fixdt(1, 18, 17)  SampleTime=7.65403750478377e-09
  Gain3_const : Constant  Value=0.019999980926513671875  OutDataTypeStr=fixdt(1, 18, 22)  SampleTime=7.65403750478377e-09
  Gain3_out1_bypass : Subsystem
  HwModeRegister : Delay  DelayLength=double(1)  InitialCondition=0  SampleTime=7.65403750478377e-09
  HwModeRegister1 : Delay  DelayLength=double(1)  InitialCondition=0  SampleTime=7.65403750478377e-09
  PipelineRegister : Delay  DelayLength=double(1)  InitialCondition=0  SampleTime=7.65403750478377e-09
  Serializer_Subnetwork : Subsystem
  Serializer_Subnetwork1 : Subsystem
  _in0_unit_delay : simulink_need_slupdate/Unit Delay Enabled  vinit=0.0  tsamp=-1
  counter : Subsystem
  enb_counter_eq_23 : simulink/Logic and Bit Operations/Compare To Constant  relop===  const=double(23)  OutDataTypeStr=boolean
  enb_counter_eq_24 : simulink/Logic and Bit Operations/Compare To Constant  relop===  const=double(24)  OutDataTypeStr=boolean
  enb_counter_le_1 : simulink/Logic and Bit Operations/Compare To Constant  relop=<=  const=double(1)  OutDataTypeStr=boolean
  mux : Mux  Inputs=2
  mux1 : Mux  Inputs=2
  nequ_dtc{,1..3} (4 alike) : DataTypeConversion  OutDataTypeStr=fixdt(1, 18, 0)  ConvertRealWorld=Stored Integer (SI)  SampleTime=7.65403750478377e-09  SaturateOnIntegerOverflow=off  RndMeth=Floor
  nequ_dtc4 : DataTypeConversion  OutDataTypeStr=fixdt(1, 36, 23)  ConvertRealWorld=Stored Integer (SI)  SampleTime=7.65403750478377e-09  SaturateOnIntegerOverflow=off  RndMeth=Floor
  nequ_dtc5 : DataTypeConversion  OutDataTypeStr=fixdt(1, 36, 28)  ConvertRealWorld=Stored Integer (SI)  SampleTime=7.65403750478377e-09  SaturateOnIntegerOverflow=off  RndMeth=Floor
  rd_0 : Delay  DelayLength=double(10)  InitialCondition=0  SampleTime=7.65403750478377e-09
  rd_{1..2,5..6} (4 alike) : Delay  DelayLength=double(1)  InitialCondition=0  SampleTime=7.65403750478377e-09
  rd_3 : Delay  DelayLength=double(29)  InitialCondition=0  SampleTime=7.65403750478377e-09
  rd_4 : Delay  DelayLength=double(29)  InitialCondition=0  SampleTime=7.65403750478377e-09
  rd_7 : Delay  DelayLength=double(10)  InitialCondition=0  SampleTime=7.65403750478377e-09
  out0 : Outport  OutDataTypeStr=fixdt(1, 36, 23)  PortDimensions=[6]  SampleTime=7.65403750478377e-09
  out1 : Outport  Port=2  OutDataTypeStr=fixdt(1, 36, 28)  PortDimensions=[6]  SampleTime=7.65403750478377e-09
  wires:
  nequ_dtc4/1 -> out0/1
  nequ_dtc5/1 -> out1/1
  _in0_unit_delay/1 -> nequ_dtc4/1
  Gain3_out1_bypass/1(out0) -> nequ_dtc5/1
  rd_6/1 -> Gain3_out1_bypass/1(in0)
  rd_7/1 -> Gain3_out1_bypass/2(in1)
  rd_0/1 -> _in0_unit_delay/2
  Gain1/1 -> PipelineRegister/1
  HwModeRegister1/1 -> Gain1/2
  HwModeRegister/1 -> Gain1/1
  rd_4/1 -> HwModeRegister1/1
  Serializer_Subnetwork/1(out0) -> HwModeRegister/1
  Serializer_Subnetwork1/1(out0) -> rd_4/1
  rd_5/1 -> _in0_unit_delay/1
  rd_3/1 -> Serializer_Subnetwork/2(in1)
  rd_1/1 -> Serializer_Subnetwork/1(in0)
  counter/1(out0) -> rd_3/1, Serializer_Subnetwork1/2(in1)
  mux1/1 -> Serializer_Subnetwork1/1(in0)
  PipelineRegister/1 -> rd_5/1, rd_6/1
  rd_2/1 -> counter/Enable
  nequ_dtc3/1 -> mux1/2
  nequ_dtc2/1 -> mux1/1
  nequ_dtc1/1 -> mux/2
  nequ_dtc/1 -> mux/1
  enb_counter_eq_23/1 -> rd_0/1
  Gain3_const/1 -> nequ_dtc3/1
  Gain1_const/1 -> nequ_dtc2/1
  in1/1 -> nequ_dtc1/1
  mux/1 -> rd_1/1
  enb_counter_le_1/1 -> rd_2/1
  in0/1 -> nequ_dtc/1
  enb_counter_eq_24/1 -> rd_7/1
  enb_counter/1 -> enb_counter_le_1/1, enb_counter_eq_24/1, enb_counter_eq_23/1

== system gm_HDL_pfc_gold_fi_vnl/simscape_system/simscape_system/HDL Subsystem/Sparse Matrix-Vector Product ==
  in0 : Inport  OutDataTypeStr=fixdt(1, 25, 13)  PortDimensions=[10]  SampleTime=7.65403750478377e-09
  selectSignal : Inport  Port=2  OutDataTypeStr=boolean  SampleTime=7.65403750478377e-09
  enb_counter : Inport  Port=3  OutDataTypeStr=fixdt(0, 7, 0)  SampleTime=7.65403750478377e-09
  SelectCols{1..6} (6 alike) : Selector  InputPortWidth=10  IndexOptions=Index vector (dialog)  Indices=double([2 3 4 5 6 7 8 9 10])  OutputSizes=double(1)
  SelectCols7 : Selector  InputPortWidth=10  IndexOptions=Index vector (dialog)  Indices=double([1 2 3 4 5 6 7 8 9])  OutputSizes=double(1)
  SelectRows1 : Selector  InputPortWidth=63  IndexOptions=Index vector (dialog)  Indices=double([2 9 16 23 30 37 44 51 58])  OutputSizes=double(1)
  SelectRows2 : Selector  InputPortWidth=63  IndexOptions=Index vector (dialog)  Indices=double([3 10 17 24 31 38 45 52 59])  OutputSizes=double(1)
  SelectRows3 : Selector  InputPortWidth=63  IndexOptions=Index vector (dialog)  Indices=double([4 11 18 25 32 39 46 53 60])  OutputSizes=double(1)
  SelectRows4 : Selector  InputPortWidth=63  IndexOptions=Index vector (dialog)  Indices=double([5 12 19 26 33 40 47 54 61])  OutputSizes=double(1)
  SelectRows5 : Selector  InputPortWidth=63  IndexOptions=Index vector (dialog)  Indices=double([6 13 20 27 34 41 48 55 62])  OutputSizes=double(1)
  SelectRows6 : Selector  InputPortWidth=63  IndexOptions=Index vector (dialog)  Indices=double([7 14 21 28 35 42 49 56 63])  OutputSizes=double(1)
  SelectRows7 : Selector  InputPortWidth=63  IndexOptions=Index vector (dialog)  Indices=double([1 8 15 22 29 36 43 50 57])  OutputSizes=double(1)
  concatenate : Concatenate  NumInputs=7
  configuration1_wire : hdlmdlgenlib/Buffer
  const : Constant  Value=[-0.000935040414333343505859375;0.00615119002759456634521484375;-0.003075595013797283172607421875;-0.003075595013797283172607421875;-0.003075600601732730865478515625;-0.003075600601732730865478515625;0.0061512016691267490386962890625;0.0004675202071666717529296875;-0.00615119002759456634521484375;0.003075595013797283172607421875;0.003075595013797283172607421875;0.003075600601732730865478515625;0.003075600601732730865478515625;-0.0061512016691267490386962890625;0.0004675202071666717529296875;0.003075595013797283172607421875;-0.00615119002759456634521484375;0.003075595013797283172607421875;-0.0061512016691267490386962890625;0.003075600601732730865478515625;0.003075600601732730865478515625;0.0004675202071666717529296875;0.003075595013797283172607421875;0.003075595013797283172607421875;-0.00615119002759456634521484375;0.003075600601732730865478515625;-0.0061512016691267490386962890625;0.003075600601732730865478515625;0.0004675202071666717529296875;-0.003075595013797283172607421875;0.00615119002759456634521484375;-0.003075595013797283172607421875;0.0061512016691267490386962890625;-0.003075600601732730865478515625;-0.003075600601732730865478515625;0.0004675202071666717529296875;-0.003075595013797283172607421875;-0.003075595013797283172607421875;0.00615119002759456634521484375;-0.003075600601732730865478515625;0.0061512016691267490386962890625;-0.003075600601732730865478515625;0.0004675202071666717529296875;0.0002460475079715251922607421875;-0.00012302398681640625;-0.00012302398681640625;-0.00012302398681640625;-0.00012302398681640625;0.0002460479736328125;0;-0.00012302398681640625;0.0002460475079715251922607421875;-0.00012302398681640625;0.0002460479736328125;-0.00012302398681640625;-0.00012302398681640625;0;-0.00012302398681640625;-0.00012302398681640625;0.0002460475079715251922607421875;-0.00012302398681640625;0.0002460479736328125;-0.00012302398681640625]  OutDataTypeStr=fixdt(1, 25, 31)  SampleTime=7.65403750478377e-09
  dtc{,1..6} (7 alike) : DataTypeConversion  OutDataTypeStr=fixdt(1, 25, 13)  RndMeth=Nearest  SampleTime=7.65403750478377e-09  SaturateOnIntegerOverflow=off
  hNNewMatrixB_shared : Subsystem
  rd_{0..12} (13 alike) : Delay  DelayLength=double(1)  InitialCondition=0  SampleTime=7.65403750478377e-09
  terminator : Terminator
  matrixBOutSignal : Outport  OutDataTypeStr=fixdt(1, 25, 13)  PortDimensions=[7]  SampleTime=7.65403750478377e-09
  wires:
  rd_12/1 -> concatenate/7
  rd_10/1 -> concatenate/6
  rd_8/1 -> concatenate/5
  concatenate/1 -> matrixBOutSignal/1
  rd_4/1 -> concatenate/3
  rd_2/1 -> concatenate/2
  dtc/1 -> concatenate/1
  dtc5/1 -> rd_10/1
  dtc3/1 -> rd_6/1
  dtc2/1 -> rd_4/1
  dtc1/1 -> rd_2/1
  rd_0/1 -> dtc/1
  rd_9/1 -> dtc5/1
  rd_7/1 -> dtc4/1
  dtc4/1 -> rd_8/1
  rd_5/1 -> dtc3/1
  rd_11/1 -> dtc6/1
  rd_3/1 -> dtc2/1
  hNNewMatrixB_shared/5(out4) -> rd_3/1
  hNNewMatrixB_shared/4(out3) -> rd_5/1
  hNNewMatrixB_shared/3(out2) -> rd_7/1
  hNNewMatrixB_shared/2(out1) -> rd_9/1
  hNNewMatrixB_shared/1(out0) -> rd_11/1
  enb_counter/1 -> hNNewMatrixB_shared/15(enb_counter)
  SelectCols1/1 -> hNNewMatrixB_shared/14(in13)
  SelectRows1/1 -> hNNewMatrixB_shared/13(in12)
  dtc6/1 -> rd_12/1
  SelectCols2/1 -> hNNewMatrixB_shared/12(in11)
  hNNewMatrixB_shared/7(out6) -> rd_0/1
  SelectRows2/1 -> hNNewMatrixB_shared/11(in10)
  SelectCols3/1 -> hNNewMatrixB_shared/10(in9)
  SelectRows3/1 -> hNNewMatrixB_shared/9(in8)
  SelectCols4/1 -> hNNewMatrixB_shared/8(in7)
  SelectRows4/1 -> hNNewMatrixB_shared/7(in6)
  SelectCols5/1 -> hNNewMatrixB_shared/6(in5)
  SelectRows5/1 -> hNNewMatrixB_shared/5(in4)
  hNNewMatrixB_shared/6(out5) -> rd_1/1
  SelectCols6/1 -> hNNewMatrixB_shared/4(in3)
  configuration1_wire/1 -> SelectRows1/1, SelectRows2/1, SelectRows6/1, SelectRows3/1, SelectRows4/1, SelectRows7/1, SelectRows5/1
  const/1 -> configuration1_wire/1
  rd_1/1 -> dtc1/1
  in0/1 -> SelectCols1/1, SelectCols2/1, SelectCols7/1, SelectCols3/1, SelectCols6/1, SelectCols4/1, SelectCols5/1
  SelectRows6/1 -> hNNewMatrixB_shared/3(in2)
  selectSignal/1 -> terminator/1
  rd_6/1 -> concatenate/4
  SelectRows7/1 -> hNNewMatrixB_shared/1(in0)
  SelectCols7/1 -> hNNewMatrixB_shared/2(in1)

== system gm_HDL_pfc_gold_fi_vnl/simscape_system/simscape_system/HDL Subsystem/Sparse Matrix-Vector Product1 ==
  delayOutSignal : Inport  OutDataTypeStr=fixdt(1, 25, 13)  PortDimensions=[7]  SampleTime=7.65403750478377e-09
  selectSignal : Inport  Port=2  OutDataTypeStr=boolean  SampleTime=7.65403750478377e-09
  enb_counter : Inport  Port=3  OutDataTypeStr=fixdt(0, 7, 0)  SampleTime=7.65403750478377e-09
  SelectCols{1..6} (6 alike) : Selector  InputPortWidth=7  IndexOptions=Index vector (dialog)  Indices=double([1 2 3 4 5 6])  OutputSizes=double(1)
  SelectCols7 : Selector  InputPortWidth=7  IndexOptions=Index vector (dialog)  Indices=double([1 2 3 4 5 7])  OutputSizes=double(1)
  SelectRows1 : Selector  InputPortWidth=42  IndexOptions=Index vector (dialog)  Indices=double([1 8 15 22 29 36])  OutputSizes=double(1)
  SelectRows2 : Selector  InputPortWidth=42  IndexOptions=Index vector (dialog)  Indices=double([2 9 16 23 30 37])  OutputSizes=double(1)
  SelectRows3 : Selector  InputPortWidth=42  IndexOptions=Index vector (dialog)  Indices=double([3 10 17 24 31 38])  OutputSizes=double(1)
  SelectRows4 : Selector  InputPortWidth=42  IndexOptions=Index vector (dialog)  Indices=double([4 11 18 25 32 39])  OutputSizes=double(1)
  SelectRows5 : Selector  InputPortWidth=42  IndexOptions=Index vector (dialog)  Indices=double([5 12 19 26 33 40])  OutputSizes=double(1)
  SelectRows6 : Selector  InputPortWidth=42  IndexOptions=Index vector (dialog)  Indices=double([6 13 20 27 34 41])  OutputSizes=double(1)
  SelectRows7 : Selector  InputPortWidth=42  IndexOptions=Index vector (dialog)  Indices=double([7 14 21 28 35 42])  OutputSizes=double(1)
  concatenate : Concatenate  NumInputs=7
  configuration1_wire : hdlmdlgenlib/Buffer
  const : Constant  Value=[0.559759318828582763671875;-0.27987849712371826171875;-0.27987849712371826171875;-0.279879033565521240234375;-0.279879033565521240234375;0.55975806713104248046875;0;-0.27987849712371826171875;0.559759318828582763671875;-0.27987849712371826171875;0.55975806713104248046875;-0.279879033565521240234375;-0.279879033565521240234375;0;-0.27987849712371826171875;-0.27987849712371826171875;0.559759318828582763671875;-0.279879033565521240234375;0.55975806713104248046875;-0.279879033565521240234375;0;-0.05037820339202880859375;0.100756466388702392578125;-0.05037820339202880859375;0.100757062435150146484375;-0.050378322601318359375;-0.050378322601318359375;0;-0.05037820339202880859375;-0.05037820339202880859375;0.100756466388702392578125;-0.050378322601318359375;0.100757062435150146484375;-0.050378322601318359375;0;0.100756466388702392578125;-0.05037820339202880859375;-0.05037820339202880859375;-0.050378322601318359375;-0.050378322601318359375;0.100757062435150146484375;0.999971926212310791015625]  OutDataTypeStr=fixdt(1, 25, 24)  SampleTime=7.65403750478377e-09
  dtc{,1..6} (7 alike) : DataTypeConversion  OutDataTypeStr=fixdt(1, 25, 13)  RndMeth=Nearest  SampleTime=7.65403750478377e-09  SaturateOnIntegerOverflow=off
  hNNewMatrixA_shared : Subsystem
  rd_{0..12} (13 alike) : Delay  DelayLength=double(1)  InitialCondition=0  SampleTime=7.65403750478377e-09
  terminator : Terminator
  matrixAOutSignal : Outport  OutDataTypeStr=fixdt(1, 25, 13)  PortDimensions=[7]  SampleTime=7.65403750478377e-09
  wires:
  rd_12/1 -> concatenate/7
  rd_10/1 -> concatenate/6
  rd_8/1 -> concatenate/5
  rd_6/1 -> concatenate/4
  rd_4/1 -> concatenate/3
  concatenate/1 -> matrixAOutSignal/1
  rd_2/1 -> concatenate/2
  dtc6/1 -> rd_12/1
  dtc3/1 -> rd_6/1
  dtc2/1 -> rd_4/1
  dtc1/1 -> rd_2/1
  rd_9/1 -> dtc5/1
  rd_7/1 -> dtc4/1
  rd_3/1 -> dtc2/1
  rd_1/1 -> dtc1/1
  hNNewMatrixA_shared/7(out6) -> rd_0/1
  hNNewMatrixA_shared/5(out4) -> rd_3/1
  dtc/1 -> concatenate/1
  hNNewMatrixA_shared/4(out3) -> rd_5/1
  hNNewMatrixA_shared/3(out2) -> rd_7/1
  hNNewMatrixA_shared/2(out1) -> rd_9/1
  hNNewMatrixA_shared/1(out0) -> rd_11/1
  enb_counter/1 -> hNNewMatrixA_shared/15(enb_counter)
  SelectRows1/1 -> hNNewMatrixA_shared/13(in12)
  SelectCols2/1 -> hNNewMatrixA_shared/12(in11)
  hNNewMatrixA_shared/6(out5) -> rd_1/1
  SelectCols3/1 -> hNNewMatrixA_shared/10(in9)
  SelectRows2/1 -> hNNewMatrixA_shared/11(in10)
  rd_11/1 -> dtc6/1
  SelectRows3/1 -> hNNewMatrixA_shared/9(in8)
  SelectCols5/1 -> hNNewMatrixA_shared/6(in5)
  rd_0/1 -> dtc/1
  SelectRows5/1 -> hNNewMatrixA_shared/5(in4)
  SelectCols6/1 -> hNNewMatrixA_shared/4(in3)
  SelectCols1/1 -> hNNewMatrixA_shared/14(in13)
  SelectCols7/1 -> hNNewMatrixA_shared/2(in1)
  SelectRows7/1 -> hNNewMatrixA_shared/1(in0)
  rd_5/1 -> dtc3/1
  dtc5/1 -> rd_10/1
  SelectRows6/1 -> hNNewMatrixA_shared/3(in2)
  delayOutSignal/1 -> SelectCols1/1, SelectCols2/1, SelectCols3/1, SelectCols4/1, SelectCols7/1, SelectCols5/1, SelectCols6/1
  const/1 -> configuration1_wire/1
  SelectCols4/1 -> hNNewMatrixA_shared/8(in7)
  dtc4/1 -> rd_8/1
  configuration1_wire/1 -> SelectRows3/1, SelectRows1/1, SelectRows4/1, SelectRows2/1, SelectRows5/1, SelectRows6/1, SelectRows7/1
  selectSignal/1 -> terminator/1
  SelectRows4/1 -> hNNewMatrixA_shared/7(in6)
